simulink model "chap7_2sim"  (Simulink 3.00)
settings: Solver=ode45  StartTime=0.0  StopTime=20  FixedStep=0.001  RelTol=1e-3  AbsTol=1e-3
settings Model: LastModifiedBy=liu

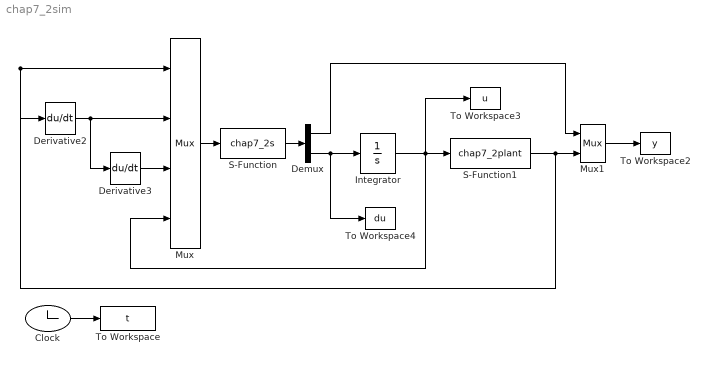
== system chap7_2sim ==
  Clock : Clock
  Demux : Demux  Outputs=2
  Derivative2 : Derivative
  Derivative3 : Derivative
  Integrator : Integrator  ExternalReset=none  InitialConditionSource=internal  InitialCondition=0  LimitOutput=off  UpperSaturationLimit=inf  LowerSaturationLimit=-inf  ShowSaturationPort=off  ShowStatePort=off  AbsoluteTolerance=auto
  Mux : Mux  Inputs=4
      settings: DisplayOption=none
  Mux1 : Mux  Inputs=2
      settings: DisplayOption=none
  S-Function : S-Function  FunctionName=chap7_2s  PortCounts=[]  SFunctionModules=''
  S-Function1 : S-Function  FunctionName=chap7_2plant  PortCounts=[]  SFunctionModules=''
  To Workspace : ToWorkspace  VariableName=t  SampleTime=-1  SaveFormat=Matrix
  To Workspace2 : ToWorkspace  VariableName=y  SampleTime=-1  SaveFormat=Matrix
  To Workspace3 : ToWorkspace  VariableName=u  SampleTime=-1  SaveFormat=Matrix
  To Workspace4 : ToWorkspace  VariableName=du  SampleTime=-1  SaveFormat=Matrix
  wires:
  Mux/1 -> S-Function/1
  S-Function/1 -> Demux/1
  Integrator/1 -> To Workspace3/1, S-Function1/1, Mux/4
  Mux1/1 -> To Workspace2/1
  S-Function1/1 -> Mux1/2, Mux/1, Derivative2/1
  Demux/1 -> Mux1/1
  Demux/2 -> Integrator/1, To Workspace4/1
  Derivative3/1 -> Mux/3
  Derivative2/1 -> Mux/2, Derivative3/1
  Clock/1 -> To Workspace/1
